simulink model "moteur2020bis"  (R2018a)
settings: Solver=VariableStepAuto  StartTime=0.0  StopTime=Tsim  RelTol=1e-3  EnableMultiTasking=on
values from neighbouring files (symbols this model uses):
  Cr = 0.02068    [moteur_bf.m]    (also in moteur_bf2.m)
  E = 50    [moteur_bf.m]    (also in moteur_bf2.m)
  f = 6.79e-5    (= 6.79e-05)    [moteur_bf.m]    (also in moteur_bf2.m)
  J = 1.37e-4    (= 0.000137)    [moteur_bf.m]    (also in moteur_bf2.m)
  k = 0.209    [moteur_bf.m]    (also in moteur_bf2.m)
  L = 1e-3    (= 0.001)    [moteur_bf.m]    (also in moteur_bf2.m)
  R = 5    [moteur_bf.m]    (also in moteur_bf2.m)
settings Model: Creator=Etudiant  LastModifiedBy=tomto
settings DataIOCC: LimitDataPoints=on
settings OptimizationCC: LifeSpan=inf
settings DebuggingCC: AllowSymbolicDim=off  SFUnexpectedBacktrackingDiag=warning  SFNoUnconditionalDefaultTransitionDiag=warning  SFExecutionAtInitializationDiag=none
settings ModelReferenceCC: PropagateSignalLabelsOutOfModel=off
settings CodeAppCC: StateflowObjectComments=on
settings GRTTargetCC: TargetLangStandard=C89/C90 (ANSI)
settings ConfigComp: CovMetricSettings=dw  CovHtmlReporting=on  CovSaveCumulativeToWorkspaceVar=on  CovSaveSingleToWorkspaceVar=on  CovExternalEMLEnable=off

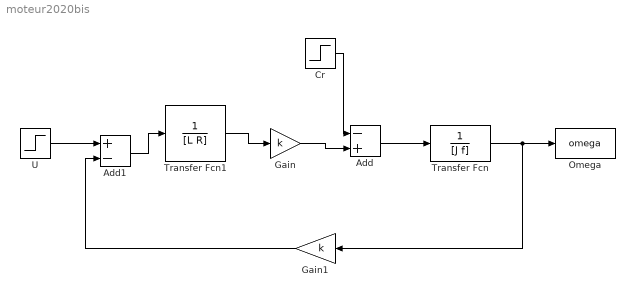
== system moteur2020bis ==
  Add : Sum  Inputs=-+
  Add1 : Sum  Inputs=+-
  Cr : Step  Time=2.5  After=Cr  SampleTime=0
  Gain : Gain  Gain=k
  Gain1 : Gain  Gain=k
  Omega : ToWorkspace  VariableName=omega  SaveFormat=Timeseries  SampleTime=-1
  Transfer Fcn : TransferFcn  Denominator=[J f]
  Transfer Fcn1 : TransferFcn  Denominator=[L R]
  U : Step  Time=0  After=E  SampleTime=0
  wires:
  U/1 -> Add1/1
  Gain1/1 -> Add1/2
  Add1/1 -> Transfer Fcn1/1
  Transfer Fcn1/1 -> Gain/1
  Gain/1 -> Add/2
  Add/1 -> Transfer Fcn/1
  Transfer Fcn/1 -> Gain1/1, Omega/1
  Cr/1 -> Add/1
